simulink model "Subsystem"  (R2020b)
settings: Solver=VariableStepAuto  StartTime=0.0  StopTime=10.0  RelTol=1e-3
settings Model: Creator=hp  LastModifiedBy=hp
settings DataIOCC: SaveOutput=off  SaveTime=off

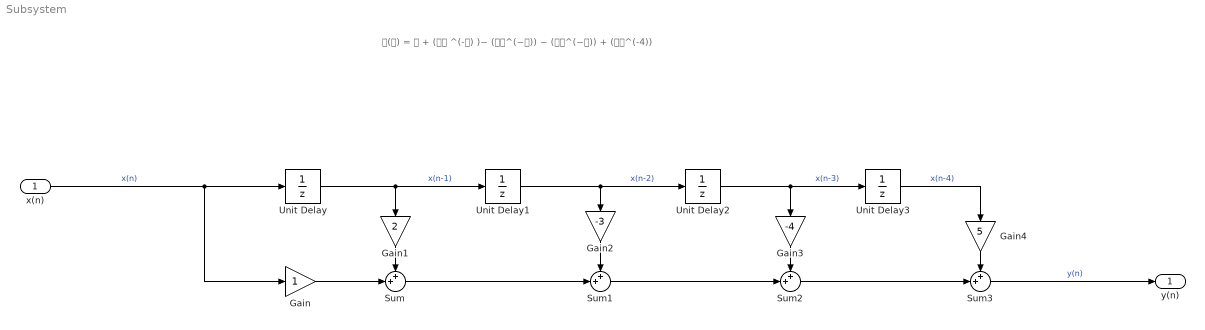
== system Subsystem ==
  note: 𝐇(𝐳) = 𝟏 + (𝟐𝐳 ^(-𝟏) )− (𝟑𝐳^(−𝟐)) − (𝟒𝐳^(−𝟑)) + (𝟓𝐳^(-4))
  x(n) : Inport  OutDataTypeStr=double  PortDimensions=1  SampleTime=0
  Gain : Gain
  Gain1 : Gain  Gain=2
  Gain2 : Gain  Gain=-3
  Gain3 : Gain  Gain=-4
  Gain4 : Gain  Gain=5
  Sum{,1..3} (4 alike) : Sum  Inputs=++|
  Unit Delay{,1..3} (4 alike) : UnitDelay  SampleTime=-1  HasFrameUpgradeWarning=on
  y(n) : Outport  OutDataTypeStr=double  PortDimensions=1  SampleTime=0
  wires:
  Unit Delay1/1 -> Gain2/1, Unit Delay2/1  "x(n-2)"
  Unit Delay/1 -> Unit Delay1/1, Gain1/1  "x(n-1)"
  Sum/1 -> Sum1/2
  Sum1/1 -> Sum2/2
  Gain2/1 -> Sum1/1
  Gain3/1 -> Sum2/1
  Unit Delay3/1 -> Gain4/1  "x(n-4)"
  Gain1/1 -> Sum/1
  Sum2/1 -> Sum3/2
  Gain4/1 -> Sum3/1
  Gain/1 -> Sum/2
  Unit Delay2/1 -> Gain3/1, Unit Delay3/1  "x(n-3)"
  x(n)/1 -> Unit Delay/1, Gain/1  "x(n)"
  Sum3/1 -> y(n)/1  "y(n)"
